simulink model "HWbridge_S_DoS"  (R2019a)
settings: Solver=ode5  StartTime=0.0  StopTime=Tf  RelTol=1e-3  EnableMultiTasking=on
values from neighbouring files (symbols this model uses):
  DoS_s = Selection(1,:)*0    [main.m]
undefined symbols (not defined in the file or in its folder): A1, AA, Ac, alph_a, alph_b, B1, BB, Bc, c0_a, c0_b, C1, Cc, D1, Dc, dtint, GG, HWbridge_data, intensity, Kdev, nloc, Ocn, Ocna, Ocnd, Ocnv, Oen, Omn, Omna, Omnd, solver, Umax, Yecm
settings Model: Creator=gutierrez-soto.1  LastModifiedBy=ferch
settings DataIOCC: MaxDataPoints=500  SaveFormat=Array  SignalLoggingSaveFormat=ModelDataLogs  SaveOutput=off  SaveTime=off  ReturnWorkspaceOutputs=off  SignalLoggingName=sigsOut
settings DebuggingCC: SaveWithParameterizedLinksMsg=none  UnderspecifiedInitializationDetection=Classic  MergeDetectMultiDrivingBlocksExec=none  SignalResolutionControl=TryResolveAllWithWarning  MultiTaskDSMMsg=warning  MultiTaskCondExecSysMsg=none  ArithmeticOperatorsInVariantConditions=warning
settings HardwareCC: ProdBitPerPointer=32  ProdBitPerSizeT=32  ProdBitPerPtrDiffT=32  ProdLargestAtomicFloat=None  ProdIntDivRoundTo=Undefined  ProdEndianess=Unspecified  ProdWordSize=32  ProdHWDeviceType=32-bit Generic  TargetUnknown=on
settings ModelReferenceCC: PropagateSignalLabelsOutOfModel=off
settings SFSimCC: SimUseLocalCustomCode=off
settings RTWCC: RTWUseLocalCustomCode=off
settings CodeAppCC: StateflowObjectComments=on
settings GRTTargetCC: TargetLangStandard=C89/C90 (ANSI)  CombineOutputUpdateFcns=off  GRTInterface=on
settings ConfigComp: CovMetricSettings=dw  CovSaveCumulativeToWorkspaceVar=on  CovSaveSingleToWorkspaceVar=on  CovExternalEMLEnable=off

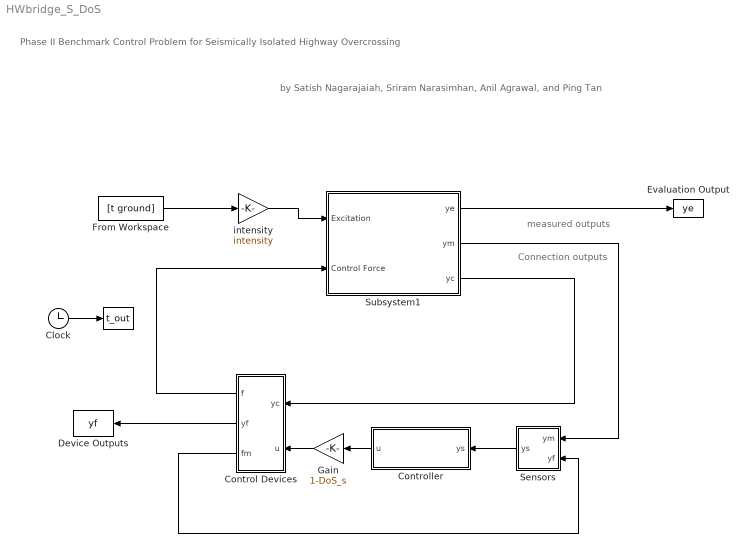
== system HWbridge_S_DoS ==
  note: by
      | Satish Nagarajaiah, Sriram Narasimhan,
      | Anil Agrawal, and Ping Tan
  note: Phase II Benchmark Control Problem for Seismically Isolated Highway Overcrossing
  note: Connection outputs
  note: measured outputs
  "    " : ToWorkspace  VariableName=t_out  SampleTime=dtint
      settings: Decimation=Num_decimate
  Clock : Clock
  Control Devices : Subsystem
  Controller : Subsystem
  Device Outputs : ToWorkspace  VariableName=yf  SampleTime=-1
      settings: Decimation=Num_decimate
  Evaluation Output : ToWorkspace  VariableName=ye  SampleTime=-1
      settings: Decimation=Num_decimate
  From Workspace : FromWorkspace  VariableName=[t ground]  SampleTime=dtint  ZeroCross=off
  Gain : Gain  Gain=1-DoS_s
  Sensors : Subsystem
  Subsystem1 : Subsystem
  intensity : Gain  Gain=intensity  SaturateOnIntegerOverflow=on  OutDataTypeStr=Inherit: Same as input  ParamDataTypeStr=Inherit: Same as input
  wires:
  Clock/1 -> "    "/1
  From Workspace/1 -> intensity/1
  intensity/1 -> Subsystem1/1(Excitation)
  Subsystem1/2(ym) -> Sensors/1(ym)
  Subsystem1/3(yc) -> Control Devices/1(yc)
  Subsystem1/1(ye) -> Evaluation Output/1
  Control Devices/1(f) -> Subsystem1/2(Control Force)
  Control Devices/3(fm) -> Sensors/2(yf)
  Controller/1(u) -> Gain/1
  Gain/1 -> Control Devices/2(u)
  Control Devices/2(yf) -> Device Outputs/1
  Sensors/1(ys) -> Controller/1(ys)

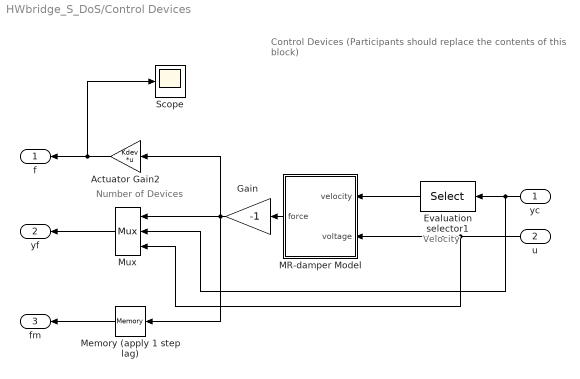
== system HWbridge_S_DoS/Control Devices ==
  note: Control Devices
      | (Participants should replace the contents of this block)
  note: Velocity
  note: Number of
      | Devices
  yc : Inport
  u : Inport  Port=2
  Actuator Gain2 : Gain  Gain=Kdev  Multiplication=Matrix(K*u)  SaturateOnIntegerOverflow=on  OutDataTypeStr=Inherit: Same as input  ParamDataTypeStr=Inherit: Same as input
  Evaluation selector1 : Selector  InputPortWidth=80  IndexOptions=Index vector (dialog)  Indices=[21:40]  OutputSizes=1
  Gain : Gain  Gain=-1  SaturateOnIntegerOverflow=on  OutDataTypeStr=Inherit: Same as input  ParamDataTypeStr=Inherit: Same as input
  MR-damper Model : Subsystem
  Memory (apply 1 step lag) : Memory  InheritSampleTime=on
  Mux : Mux  Inputs=3
  Scope : Scope
  f : Outport  InitialOutput=0
  yf : Outport  Port=2  InitialOutput=0
  fm : Outport  Port=3  InitialOutput=0
  wires:
  u/1 -> Mux/3, MR-damper Model/2(voltage)
  Evaluation selector1/1 -> MR-damper Model/1(velocity)
  Gain/1 -> Mux/1, Actuator Gain2/1, Memory (apply 1 step lag)/1
  Actuator Gain2/1 -> Scope/1, f/1
  MR-damper Model/1(force) -> Gain/1
  yc/1 -> Mux/2, Evaluation selector1/1
  Mux/1 -> yf/1
  Memory (apply 1 step lag)/1 -> fm/1

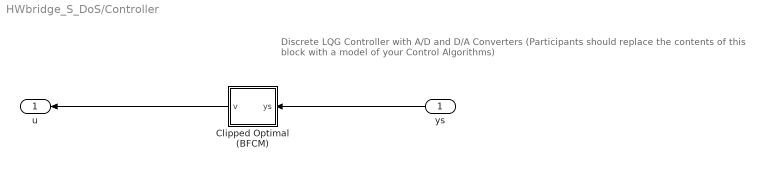
== system HWbridge_S_DoS/Controller ==
  note: Discrete LQG Controller with A/D and D/A Converters
      | (Participants should replace the contents of this block with a model of your Control Algorithms)
  ys : Inport
  Clipped Optimal (BFCM) : Subsystem
  u : Outport
  wires:
  ys/1 -> Clipped Optimal (BFCM)/1(ys)
  Clipped Optimal (BFCM)/1(v) -> u/1

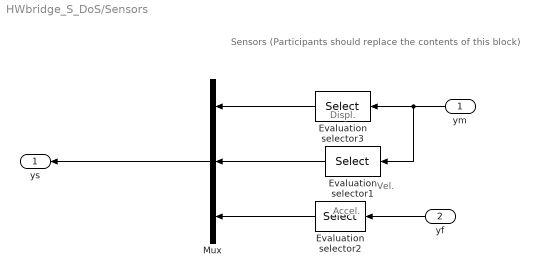
== system HWbridge_S_DoS/Sensors ==
  note: Sensors
      | (Participants should replace the contents of this block)
  note: Accel.
  note: Displ.
  note: Vel.
  ym : Inport
  yf : Inport  Port=2
  Evaluation selector1 : Selector  InputPortWidth=length(Omn)  IndexOptions=Index vector (dialog)  Indices=Omna  OutputSizes=1
  Evaluation selector2 : Selector  InputPortWidth=nloc  IndexOptions=Index vector (dialog)  Indices=1:nloc  OutputSizes=1
  Evaluation selector3 : Selector  InputPortWidth=length(Omn)  IndexOptions=Index vector (dialog)  Indices=Omnd  OutputSizes=1
  Mux : Mux  Inputs=3
  ys : Outport
  wires:
  yf/1 -> Evaluation selector2/1
  Mux/1 -> ys/1
  Evaluation selector3/1 -> Mux/1
  Evaluation selector1/1 -> Mux/2
  Evaluation selector2/1 -> Mux/3
  ym/1 -> Evaluation selector1/1, Evaluation selector3/1

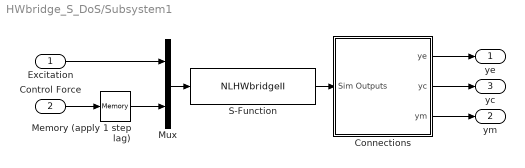
== system HWbridge_S_DoS/Subsystem1 ==
  Excitation : Inport
  Control Force : Inport  Port=2
  Connections : Subsystem
  Memory (apply 1 step lag) : Memory  InheritSampleTime=on
  Mux : Mux  Inputs=2
  S-Function : S-Function  FunctionName=NLHWbridgeII  Parameters=HWbridge_data,solver,Yecm  SFunctionDeploymentMode=off  EnableBusSupport=off
  ye : Outport
  ym : Outport  Port=2
  yc : Outport  Port=3
  wires:
  Mux/1 -> S-Function/1
  S-Function/1 -> Connections/1(Sim Outputs)
  Excitation/1 -> Mux/1
  Control Force/1 -> Memory (apply 1 step lag)/1
  Memory (apply 1 step lag)/1 -> Mux/2
  Connections/1(ye) -> ye/1
  Connections/2(yc) -> yc/1
  Connections/3(ym) -> ym/1

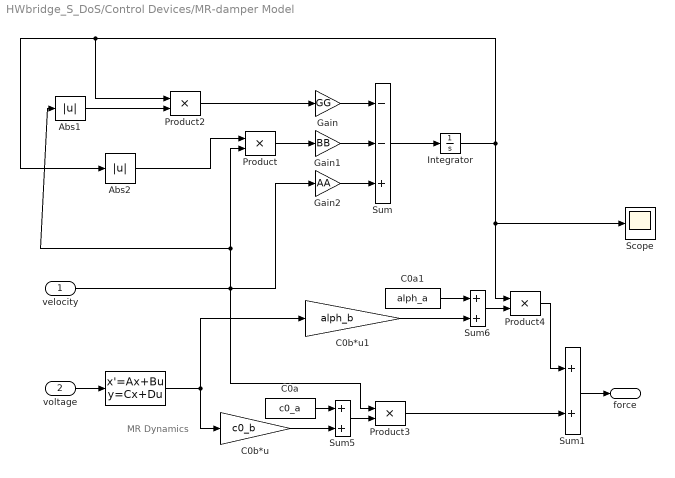
== system HWbridge_S_DoS/Control Devices/MR-damper Model ==
  note: MR Dynamics
  velocity : Inport
  voltage : Inport  Port=2
  " " : StateSpace  A=A1  B=B1  C=C1  D=D1  InitialCondition=0
  Abs1 : Abs  SaturateOnIntegerOverflow=on
  Abs2 : Abs  SaturateOnIntegerOverflow=on
  C0a : Constant  Value=c0_a
  C0a1 : Constant  Value=alph_a
  C0b*u : Gain  Gain=c0_b  SaturateOnIntegerOverflow=on  OutDataTypeStr=Inherit: Same as input  ParamDataTypeStr=Inherit: Same as input
  C0b*u1 : Gain  Gain=alph_b  SaturateOnIntegerOverflow=on  OutDataTypeStr=Inherit: Same as input  ParamDataTypeStr=Inherit: Same as input
  Gain : Gain  Gain=GG  SaturateOnIntegerOverflow=on  OutDataTypeStr=Inherit: Same as input  ParamDataTypeStr=Inherit: Same as input
  Gain1 : Gain  Gain=BB  SaturateOnIntegerOverflow=on  OutDataTypeStr=Inherit: Same as input  ParamDataTypeStr=Inherit: Same as input
  Gain2 : Gain  Gain=AA  SaturateOnIntegerOverflow=on  OutDataTypeStr=Inherit: Same as input  ParamDataTypeStr=Inherit: Same as input
  Integrator : Integrator
  Product{,2..4} (4 alike) : Product  InputSameDT=on  SaturateOnIntegerOverflow=on  OutDataTypeStr=Inherit: Same as first input
  Scope : Scope
  Sum : Sum  Inputs=--+  InputSameDT=on  SaturateOnIntegerOverflow=on  OutDataTypeStr=Inherit: Same as first input
  Sum1 : Sum  InputSameDT=on  SaturateOnIntegerOverflow=on  OutDataTypeStr=Inherit: Same as first input
  Sum5 : Sum  InputSameDT=on  SaturateOnIntegerOverflow=on  OutDataTypeStr=Inherit: Same as first input
  Sum6 : Sum  InputSameDT=on  SaturateOnIntegerOverflow=on  OutDataTypeStr=Inherit: Same as first input
  force : Outport  InitialOutput=0
  wires:
  voltage/1 -> " "/1
  " "/1 -> C0b*u1/1, C0b*u/1
  Sum1/1 -> force/1
  Abs2/1 -> Product/1
  Product2/1 -> Gain/1
  Sum/1 -> Integrator/1
  Gain/1 -> Sum/1
  Gain1/1 -> Sum/2
  Gain2/1 -> Sum/3
  Product/1 -> Gain1/1
  Abs1/1 -> Product2/2
  velocity/1 -> Product/2, Abs1/1, Gain2/1, Product3/1
  Sum5/1 -> Product3/2
  C0a/1 -> Sum5/1
  C0b*u/1 -> Sum5/2
  Sum6/1 -> Product4/2
  C0a1/1 -> Sum6/1
  C0b*u1/1 -> Sum6/2
  Product3/1 -> Sum1/2
  Product4/1 -> Sum1/1
  Integrator/1 -> Abs2/1, Product2/1, Product4/1, Scope/1

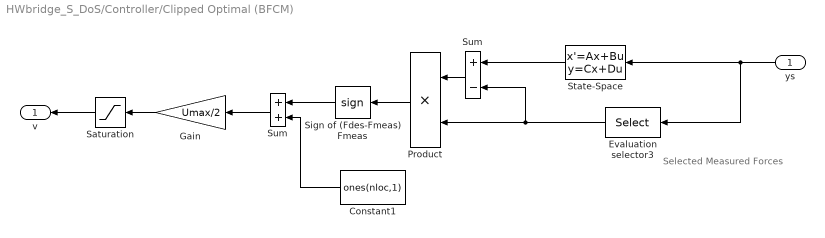
== system HWbridge_S_DoS/Controller/Clipped Optimal (BFCM) ==
  note: Selected Measured Forces
  ys : Inport
  Constant1 : Constant  Value=ones(nloc,1)
  Evaluation selector3 : Selector  InputPortWidth=36  IndexOptions=Index vector (dialog)  Indices=17:36  OutputSizes=1
  Gain : Gain  Gain=Umax/2  SaturateOnIntegerOverflow=on  OutDataTypeStr=Inherit: Same as input  ParamDataTypeStr=Inherit: Same as input
  Product : Product  InputSameDT=on  SaturateOnIntegerOverflow=on  OutDataTypeStr=Inherit: Same as first input
  Saturation : Saturate  UpperLimit=Umax  LowerLimit=-Umax
  Sign of (Fdes-Fmeas)Fmeas : Signum
  State-Space : StateSpace  A=Ac  B=Bc  C=Cc  D=Dc  InitialCondition=0
  Sum : Sum  Inputs=+-  InputSameDT=on  SaturateOnIntegerOverflow=on  OutDataTypeStr=Inherit: Same as first input
  "Sum " : Sum  InputSameDT=on  SaturateOnIntegerOverflow=on  OutDataTypeStr=Inherit: Same as first input
  v : Outport  InitialOutput=0
  wires:
  Saturation/1 -> v/1
  Evaluation selector3/1 -> Sum/2, Product/2
  ys/1 -> State-Space/1, Evaluation selector3/1
  Gain/1 -> Saturation/1
  State-Space/1 -> Sum/1
  "Sum "/1 -> Gain/1
  Constant1/1 -> "Sum "/2
  Sign of (Fdes-Fmeas)Fmeas/1 -> "Sum "/1
  Sum/1 -> Product/1
  Product/1 -> Sign of (Fdes-Fmeas)Fmeas/1

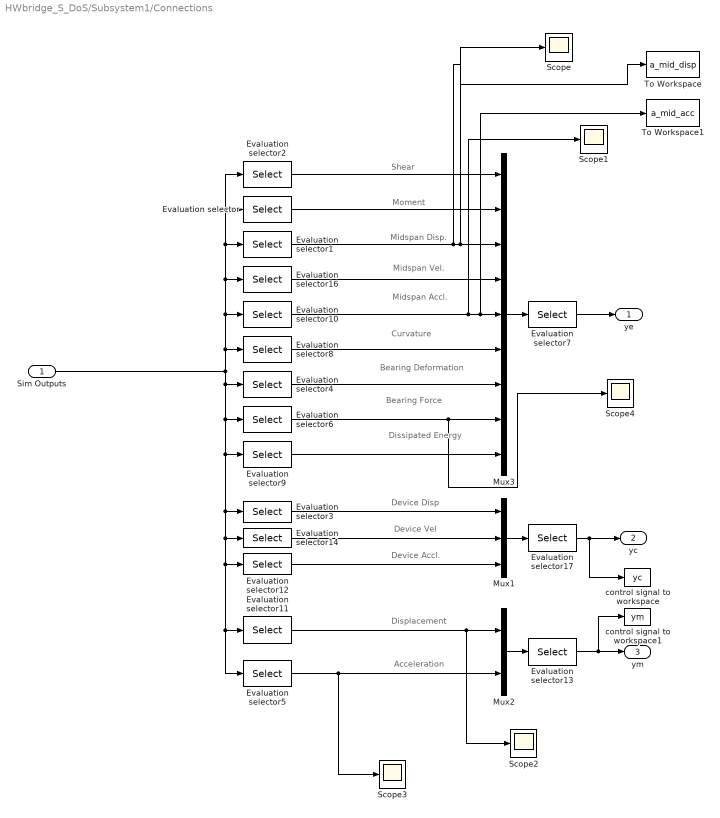
== system HWbridge_S_DoS/Subsystem1/Connections ==
  note: Acceleration
  note: Displacement
  note: Moment
  note: Bearing Deformation
  note: Device Disp
  note: Midspan Disp.
  note: Midspan Accl.
  note: Curvature
  note: Device Accl.
  note: Bearing Force
  note: Dissipated Energy
  note: Midspan Vel.
  note: Shear
  note: Device Vel
  Sim Outputs : Inport
  Evaluation selector : Selector  InputPortWidth=Oecm  IndexOptions=Index vector (dialog)  Indices=Oen_ovm  OutputSizes=1
  Evaluation selector1 : Selector  InputPortWidth=Oecm  IndexOptions=Index vector (dialog)  Indices=Oen_msd  OutputSizes=1
  Evaluation selector10 : Selector  InputPortWidth=Oecm  IndexOptions=Index vector (dialog)  Indices=Oen_msa  OutputSizes=1
  Evaluation selector11 : Selector  InputPortWidth=Oecm  IndexOptions=Index vector (dialog)  Indices=Omn(Omnd)  OutputSizes=1
  Evaluation selector12 : Selector  InputPortWidth=Oecm  IndexOptions=Index vector (dialog)  Indices=Ocn(Ocna)  OutputSizes=1
  Evaluation selector13 : Selector  InputPortWidth=length(Omn)  IndexOptions=Index vector (dialog)  Indices=1:length(Omn)  OutputSizes=1
  Evaluation selector14 : Selector  InputPortWidth=Oecm  IndexOptions=Index vector (dialog)  Indices=Ocn(Ocnv)  OutputSizes=1
  Evaluation selector16 : Selector  InputPortWidth=Oecm  IndexOptions=Index vector (dialog)  Indices=Oen_msv  OutputSizes=1
  Evaluation selector17 : Selector  InputPortWidth=length(Ocn)  IndexOptions=Index vector (dialog)  Indices=1:length(Ocn)  OutputSizes=1
  Evaluation selector2 : Selector  InputPortWidth=Oecm  IndexOptions=Index vector (dialog)  Indices=Oen_bsf  OutputSizes=1
  Evaluation selector3 : Selector  InputPortWidth=Oecm  IndexOptions=Index vector (dialog)  Indices=Ocn(Ocnd)  OutputSizes=1
  Evaluation selector4 : Selector  InputPortWidth=Oecm  IndexOptions=Index vector (dialog)  Indices=Oen_brd  OutputSizes=1
  Evaluation selector5 : Selector  InputPortWidth=Oecm  IndexOptions=Index vector (dialog)  Indices=Omn(Omna)  OutputSizes=1
  Evaluation selector6 : Selector  InputPortWidth=Oecm  IndexOptions=Index vector (dialog)  Indices=Oen_brf  OutputSizes=1
  Evaluation selector7 : Selector  InputPortWidth=length(Oen)  IndexOptions=Index vector (dialog)  Indices=Oen  OutputSizes=1
  Evaluation selector8 : Selector  InputPortWidth=Oecm  IndexOptions=Index vector (dialog)  Indices=Oen_cur  OutputSizes=1
  Evaluation selector9 : Selector  InputPortWidth=Oecm  IndexOptions=Index vector (dialog)  Indices=Oen_eng  OutputSizes=1
  Mux1 : Mux  Inputs=3
  Mux2 : Mux  Inputs=2
  Mux3 : Mux  Inputs=9
  Scope{,1..4} (5 alike) : Scope
  To Workspace : ToWorkspace  VariableName=a_mid_disp  SaveFormat=Timeseries  SampleTime=-1
  To Workspace1 : ToWorkspace  VariableName=a_mid_acc  SaveFormat=Timeseries  SampleTime=-1
  control signal to workspace : ToWorkspace  VariableName=yc  SampleTime=-1
      settings: Decimation=Num_decimate
  control signal to workspace1 : ToWorkspace  VariableName=ym  SampleTime=-1
      settings: Decimation=Num_decimate
  ye : Outport
  yc : Outport  Port=2
  ym : Outport  Port=3
  wires:
  Mux2/1 -> Evaluation selector13/1
  Evaluation selector5/1 -> Scope3/1, Mux2/2
  Evaluation selector11/1 -> Scope2/1, Mux2/1
  Evaluation selector13/1 -> ym/1, control signal to workspace1/1
  Mux3/1 -> Evaluation selector7/1
  Evaluation selector14/1 -> Mux1/2
  Mux1/1 -> Evaluation selector17/1
  Evaluation selector3/1 -> Mux1/1
  Evaluation selector17/1 -> yc/1, control signal to workspace/1
  Evaluation selector7/1 -> ye/1
  Evaluation selector2/1 -> Mux3/1
  Evaluation selector/1 -> Mux3/2
  Evaluation selector1/1 -> To Workspace/1, Scope/1, Mux3/3
  Evaluation selector16/1 -> Mux3/4
  Evaluation selector10/1 -> Scope1/1, To Workspace1/1, Mux3/5
  Evaluation selector9/1 -> Mux3/9
  Evaluation selector6/1 -> Scope4/1, Mux3/8
  Evaluation selector4/1 -> Mux3/7
  Evaluation selector8/1 -> Mux3/6
  Sim Outputs/1 -> Evaluation selector4/1, Evaluation selector9/1, Evaluation selector14/1, Evaluation selector11/1, Evaluation selector5/1, Evaluation selector12/1, Evaluation selector3/1, Evaluation selector6/1, Evaluation selector1/1, Evaluation selector/1, Evaluation selector2/1, Evaluation selector16/1, Evaluation selector10/1, Evaluation selector8/1
  Evaluation selector12/1 -> Mux1/3
